simulink model "Regler_Mantel"  (R2017b)
settings: Solver=VariableStepAuto  StartTime=0.0  StopTime=44  RelTol=1e-3
values from neighbouring files (symbols this model uses):
  Kp_M = (0.35/K_Mantel)*(T1_Mantel/Tu)    (= 1.76744186047)    [Regler_Kaskadierung.m]    (also in Regler_Kaskadierung_2.m = 5; Regler_Kaskadierung_2_editor.m = 5; Regler_Mantel.m = (0.35/K_Mantel)*(T1_Mantel/Tu))
libraries: cstblocks x1
settings Model: Creator=arbno  LastModifiedBy=arbno

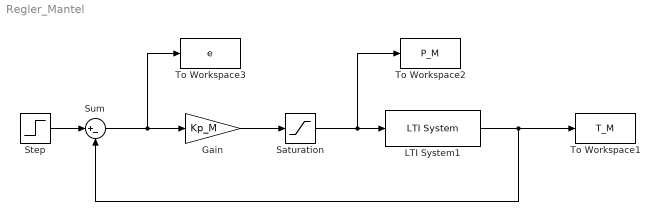
== system Regler_Mantel ==
  Gain : Gain  Gain=Kp_M
  LTI System1 : cstblocks/LTI System  sys=G_Z_Mantel  IC=[]
  Saturation : Saturate  UpperLimit=1  LowerLimit=0
  Step : Step  Time=0  SampleTime=0
  Sum : Sum  Inputs=|+-
  To Workspace1 : ToWorkspace  VariableName=T_M  SaveFormat=Structure With Time  SampleTime=-1
  To Workspace2 : ToWorkspace  VariableName=P_M  SaveFormat=Structure With Time  SampleTime=-1
  To Workspace3 : ToWorkspace  VariableName=e  SaveFormat=Structure With Time  SampleTime=-1
  wires:
  LTI System1/1 -> To Workspace1/1, Sum/2
  Step/1 -> Sum/1
  Gain/1 -> Saturation/1
  Sum/1 -> To Workspace3/1, Gain/1
  Saturation/1 -> To Workspace2/1, LTI System1/1
